simulink model "exp6_diagrama"  (R2020b)
settings: Solver=VariableStepAuto  StartTime=0.0  StopTime=10  RelTol=1e-3
values from neighbouring files (symbols this model uses):
  DC_PRBS = 4    [script_exp6.m]
  gain_PRBS = 10    [script_exp6.m]
  h = 1e-2    (= 0.01)    [script_exp6.m]
  h_motor = h*1e-3    (= 1e-05)    [script_exp6.m]
  x0 = [1;0]    [script_exp6.m]
undefined symbols (not defined in the file or in its folder): A, B, C, Ka, Kg, Kt, sigbuilder_block
libraries: simulink x4
settings Model: Creator=gusta  LastModifiedBy=lucas
settings DebuggingCC: SFMachineParentedDataDiag=error

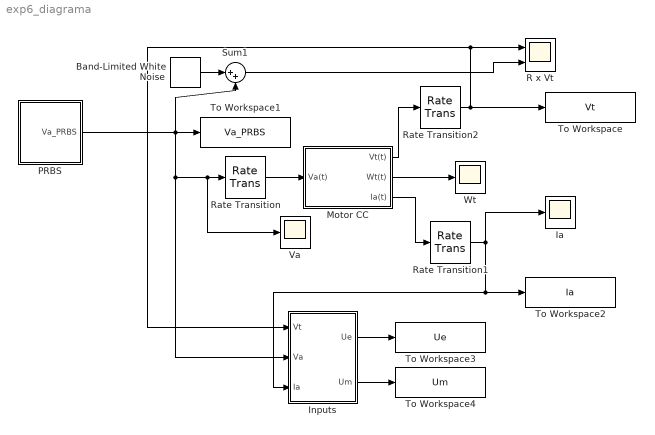
== system exp6_diagrama ==
  Band-Limited White Noise : simulink/Sources/Band-Limited White Noise  Cov=noise_power  Ts=h  seed=[23341]
  Ia : Scope
  Inputs : Subsystem
  Motor CC : Subsystem
  PRBS : Subsystem
  R x Vt : Scope  NumInputPorts=2
  Rate Transition : RateTransition  OutPortSampleTime=h_motor
  Rate Transition1 : RateTransition  OutPortSampleTime=h
  Rate Transition2 : RateTransition  OutPortSampleTime=h
  Sum1 : Sum  Inputs=|++
  To Workspace : ToWorkspace  VariableName=Vt  SaveFormat=Structure With Time  SampleTime=-1
  To Workspace1 : ToWorkspace  VariableName=Va_PRBS  SaveFormat=Structure With Time  SampleTime=-1
  To Workspace2 : ToWorkspace  VariableName=Ia  SaveFormat=Structure With Time  SampleTime=-1
  To Workspace3 : ToWorkspace  VariableName=Ue  SaveFormat=Structure With Time  SampleTime=-1
  To Workspace4 : ToWorkspace  VariableName=Um  SaveFormat=Structure With Time  SampleTime=-1
  Va : Scope
  Wt : Scope
  wires:
  Motor CC/3(Ia(t)) -> Rate Transition1/1
  Sum1/1 -> R x Vt/2
  Band-Limited White Noise/1 -> Sum1/1
  Rate Transition/1 -> Motor CC/1(Va(t))
  Rate Transition1/1 -> To Workspace2/1, Inputs/3(Ia), Ia/1
  Motor CC/1(Vt(t)) -> Rate Transition2/1
  Rate Transition2/1 -> Inputs/1(Vt), R x Vt/1, To Workspace/1
  Inputs/1(Ue) -> To Workspace3/1
  Inputs/2(Um) -> To Workspace4/1
  Motor CC/2(Wt(t)) -> Wt/1
  PRBS/1(Va_PRBS) -> Sum1/2, To Workspace1/1, Inputs/2(Va), Va/1, Rate Transition/1

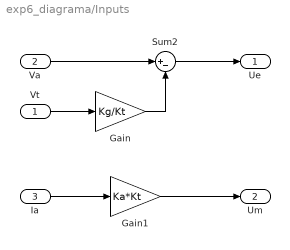
== system exp6_diagrama/Inputs ==
  Vt : Inport
  Va : Inport  Port=2
  Ia : Inport  Port=3
  Gain : Gain  Gain=Kg/Kt
  Gain1 : Gain  Gain=Ka*Kt
  Sum2 : Sum  Inputs=|+-
  Ue : Outport
  Um : Outport  Port=2
  wires:
  Gain/1 -> Sum2/2
  Gain1/1 -> Um/1
  Vt/1 -> Gain/1
  Va/1 -> Sum2/1
  Sum2/1 -> Ue/1
  Ia/1 -> Gain1/1

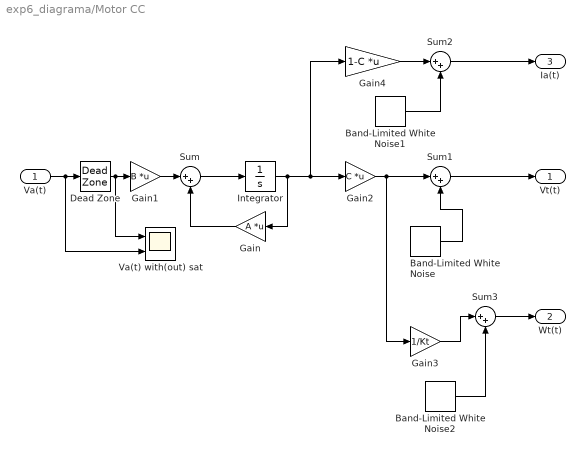
== system exp6_diagrama/Motor CC ==
  Va(t) : Inport
  Band-Limited White Noise : simulink/Sources/Band-Limited White Noise  Cov=noise_power  Ts=h_motor  seed=[23341]
  Band-Limited White Noise1 : simulink/Sources/Band-Limited White Noise  Cov=noise_power  Ts=h_motor  seed=[23341]
  Band-Limited White Noise2 : simulink/Sources/Band-Limited White Noise  Cov=noise_power  Ts=h_motor  seed=[23341]
  Dead Zone : DeadZone  LowerValue=0  UpperValue=0  SaturateOnIntegerOverflow=on
  Gain : Gain  Gain=A  Multiplication=Matrix(K*u)
  Gain1 : Gain  Gain=B  Multiplication=Matrix(K*u)
  Gain2 : Gain  Gain=C  Multiplication=Matrix(K*u)
  Gain3 : Gain  Gain=1/Kt
  Gain4 : Gain  Gain=1-C  Multiplication=Matrix(K*u)
  Integrator : Integrator  InitialCondition=x0
  Sum{,1..3} (4 alike) : Sum  Inputs=|++
  Va(t) with(out) sat : Scope  NumInputPorts=2
  Vt(t) : Outport
  Wt(t) : Outport  Port=2
  Ia(t) : Outport  Port=3
  wires:
  Sum/1 -> Integrator/1
  Integrator/1 -> Gain4/1, Gain2/1, Gain/1
  Gain2/1 -> Sum1/1, Gain3/1
  Gain1/1 -> Sum/1
  Gain/1 -> Sum/2
  Va(t)/1 -> Va(t) with(out) sat/2, Dead Zone/1
  Dead Zone/1 -> Va(t) with(out) sat/1, Gain1/1
  Sum1/1 -> Vt(t)/1
  Band-Limited White Noise/1 -> Sum1/2
  Sum2/1 -> Ia(t)/1
  Gain4/1 -> Sum2/1
  Sum3/1 -> Wt(t)/1
  Band-Limited White Noise1/1 -> Sum2/2
  Band-Limited White Noise2/1 -> Sum3/2
  Gain3/1 -> Sum3/1

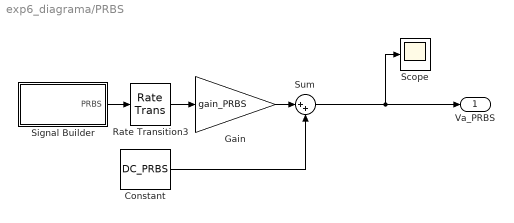
== system exp6_diagrama/PRBS ==
  Constant : Constant  Value=DC_PRBS
  Gain : Gain  Gain=gain_PRBS
  Rate Transition3 : RateTransition  OutPortSampleTime=h
  Scope : Scope
  Signal Builder : Subsystem  Tag=STV Subsys  LoadFcn=sigbuilder_block('load');  StartFcn=sigbuilder_block('start');  StopFcn=sigbuilder_block('stop');  ClipboardFcn=sigbuilder_block('clipboard');  mask(Sigbuilder block){tuvar=[0:10]}
      mask help: Simulink:masks:SigbuilderBlock_MD
      mask init:
      | if ~strcmp(get_param(bdroot(gcbh),'SimulationStatus'),'stopped') tuvar = sigbuilder_block('maskInit'); end
      settings: CopyFcn=sigbuilder_block('copy');  DeleteFcn=sigbuilder_block('delete');  ModelCloseFcn=sigbuilder_block('modelClose');  PreSaveFcn=sigbuilder_block('preSave');  PauseFcn=sigbuilder_block('pause');  ContinueFcn=sigbuilder_block('continue');  NameChangeFcn=sigbuilder_block('namechange');  OpenFcn=sigbuilder_block('open',[437.6 199.2 550.4 400 ]);  CloseFcn=sigbuilder_block('close');
      mask Display: plot(0, 0, 100, 100,[2, 2, 32, 32, 2], [68, 8, 8, 68, 68],[32, 2], [38, 38], [32, 19, 2],[53, 60, 44], [32, 17, 17, 2],[16, 16, 31, 31]);txt = getActiveGroup(gcbh);text(2, 100, txt,'verticalAlignment', 'top');
  Sum : Sum  Inputs=|++
  Va_PRBS : Outport
  wires:
  Sum/1 -> Scope/1, Va_PRBS/1
  Signal Builder/1(PRBS) -> Rate Transition3/1
  Constant/1 -> Sum/2
  Rate Transition3/1 -> Gain/1
  Gain/1 -> Sum/1

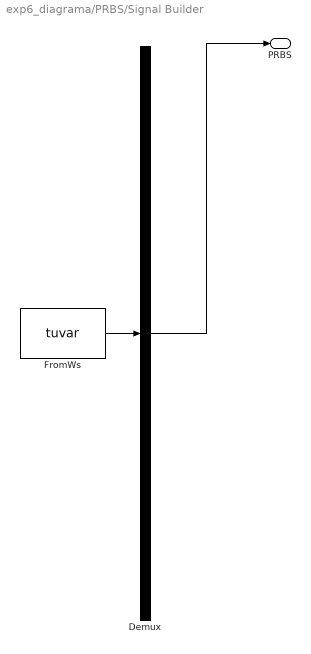
== system exp6_diagrama/PRBS/Signal Builder ==
  Demux : Demux  Tag=STV Demux  Outputs=1
      settings: DisplayOption=none
  FromWs : FromWorkspace  Tag=STV FromWs  VariableName=tuvar
      SigBuilderData=|
      | common.afterFinalStr = 'Extrapolate'
      | common.sampleTime = 0
      | dataSet.timeRange = [0 10]
      | dataSet.name = 'PRBS'
      | sbobj.Groups.Name = 'PRBS'
      | sbobj.Groups.Signals.Name = 'PRBS'
      | sbobj.Groups.Signals.XData = [0 1 1 1.5 1.5 3.5 3.5 5 5 6 6 6.5 6.5 10 10]
      | sbobj.Groups.Signals.YData = [1 1 0 0 1 1 0 0 1 1 0 0 1 1 0]
  PRBS : Outport  Tag=STV Outport
  wires:
  FromWs/1 -> Demux/1
  Demux/1 -> PRBS/1
